simulink model "freq_thruster"  (Simulink 6.0)
settings: Solver=ode4  StartTime=0.0  StopTime=2*cycles*pi/frtest  FixedStep=0.01  RelTol=1e-4
values from neighbouring files (symbols this model uses):
  cycles = 100    [MAKE25.M]
  frtest = w(i)    [bode_fit_general.m]
undefined symbols (not defined in the file or in its folder): nmiss
libraries: rov_design_analysis x1, simulink_extras x1
settings Model: Creator=john  LastModifiedBy=c  ExtModeTrigMode=oneshot  ExtModeArmWhenConnect=off
settings DataIOCC: LimitDataPoints=off
settings OptimizationCC: BooleanDataType=off
settings DebuggingCC: SolverPrmCheckMsg=none
settings HardwareCC: TargetUnknown=on

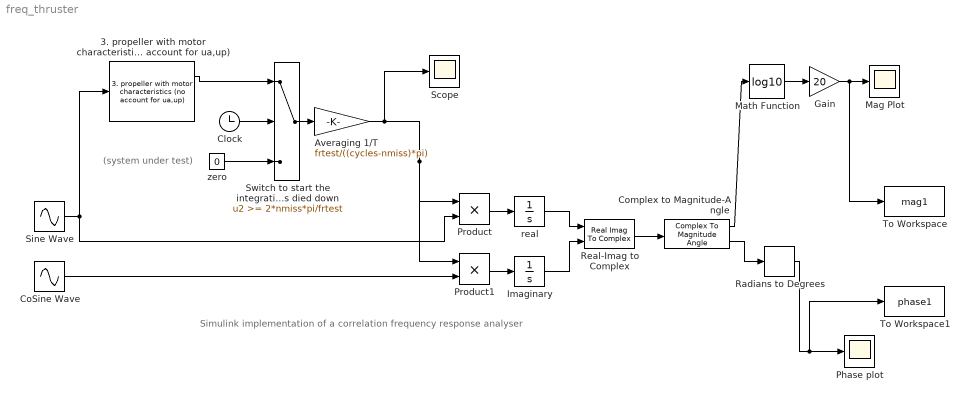
== system freq_thruster ==
  note: Simulink implementation of a correlation frequency response analyser
  note: (system under test)
  3. propeller with motor characteristics  (no account for ua,up) : rov_design_analysis/Propeller Models/3. propeller with motor characteristics  (no account for ua,up)
  "Averaging 1/T " : Gain  Gain=frtest/((cycles-nmiss)*pi)  SaturateOnIntegerOverflow=on
  Clock : Clock
  CoSine Wave : Sin  Frequency=frtest  Phase=pi/2  SampleTime=0
  Complex to Magnitude-Angle : ComplexToMagnitudeAngle
  Gain : Gain  Gain=20  SaturateOnIntegerOverflow=on
  Imaginary : Integrator
  Mag Plot : Scope
      settings: TimeRange=60  YMin=-4.1  YMax=-3.6
  Math Function : Math  Operator=log10  SaturateOnIntegerOverflow=on
  Phase plot : Scope
      settings: TimeRange=60  YMin=-250  YMax=-25
  Product : Product  SaturateOnIntegerOverflow=on  RndMeth=Zero  InputSameDT=on
  Product1 : Product  SaturateOnIntegerOverflow=on  RndMeth=Zero  InputSameDT=on
  Radians to Degrees : simulink_extras/Transformations/Radians to Degrees
  Real-Imag to Complex : RealImagToComplex
  Scope : Scope
      settings: TimeRange=60  YMin=0  YMax=0.08
  Sine Wave : Sin  Frequency=frtest  SampleTime=0
  Switch to start the integration after the transient has died down : Switch  Threshold=2*nmiss*pi/frtest  SaturateOnIntegerOverflow=on  InputSameDT=on
  To Workspace : ToWorkspace  VariableName=mag1  SampleTime=-1  SaveFormat=Array
  To Workspace1 : ToWorkspace  VariableName=phase1  SampleTime=-1  SaveFormat=Array
  real : Integrator
  zero : Constant  Value=0
  wires:
  Sine Wave/1 -> Product/2, 3. propeller with motor characteristics  (no account for ua,up)/1
  Product1/1 -> Imaginary/1
  CoSine Wave/1 -> Product1/2
  Product/1 -> real/1
  Switch to start the integration after the transient has died down/1 -> "Averaging 1/T "/1
  "Averaging 1/T "/1 -> Product/1, Product1/1, Scope/1
  real/1 -> Real-Imag to Complex/1
  Imaginary/1 -> Real-Imag to Complex/2
  Real-Imag to Complex/1 -> Complex to Magnitude-Angle/1
  Math Function/1 -> Gain/1
  Complex to Magnitude-Angle/2 -> Radians to Degrees/1
  Complex to Magnitude-Angle/1 -> Math Function/1
  3. propeller with motor characteristics  (no account for ua,up)/1 -> Switch to start the integration after the transient has died down/1
  zero/1 -> Switch to start the integration after the transient has died down/3
  Clock/1 -> Switch to start the integration after the transient has died down/2
  Gain/1 -> Mag Plot/1, To Workspace/1
  Radians to Degrees/1 -> Phase plot/1, To Workspace1/1
